simulink model "Primary_Arduino"  (R2018b)
settings: Solver=FixedStepAuto  StartTime=0  StopTime=300  MaxStep=0.01  RelTol=1e-4  EnableMultiTasking=on
libraries: pil_lib x1
settings Model: DataDictionary=data.sldd  Creator=Aliak  LastModifiedBy=Aliak
settings SolverCC: SolverResetMethod=Robust  MinimalZcImpactIntegration=on
settings OptimizationCC: DefaultParameterBehavior=Inlined  UseDivisionForNetSlopeComputation=on  UseFloatMulNetSlope=on  DefaultUnderspecifiedDataType=single  UseSpecifiedMinMax=on  InlineInvariantSignals=on  EnhancedBackFolding=on  BooleansAsBitfields=on  PassReuseOutputArgsAs=Individual arguments  StateBitsets=on  DataBitsets=on  ZeroExternalMemoryAtStartup=off  ZeroInternalMemoryAtStartup=off  NoFixptDivByZeroProtection=on  EfficientFloat2IntCast=on  LifeSpan=0.01  MaxStackSize=64  SimCompilerOptimization=on  OptimizeBlockOrder=speed  DifferentSizesBufferReuse=on
settings DebuggingCC: ConsistencyChecking=warning  ReadBeforeWriteMsg=DisableAll  WriteAfterWriteMsg=DisableAll  WriteAfterReadMsg=DisableAll  SolverPrmCheckMsg=warning  ParameterTunabilityLossMsg=error  UniqueDataStoreMsg=error  BusObjectLabelMismatch=error  StateNameClashWarn=warning  ForceCombineOutputUpdateInSim=on
settings HardwareCC: ProdBitPerInt=16  ProdBitPerPointer=16  ProdBitPerSizeT=16  ProdBitPerPtrDiffT=16  ProdLargestAtomicFloat=None  ProdWordSize=8  ProdLongLongMode=on  ProdHWDeviceType=Atmel->AVR
settings ModelReferenceCC: UpdateModelReferenceTargets=IfOutOfDate  EnableParallelModelReferenceBuilds=on  ModelReferenceMinAlgLoopOccurrences=on
settings SFSimCC: SimUserIncludeDirs="\"nativelibs/include\" \"nativelibs/src\" \"nativelibs/build\""  SFSimEcho=off  MATLABDynamicMemAlloc=off
settings RTWCC: SystemTargetFile=ert.tlc  HardwareBoard=Arduino Uno  TemplateMakefile=ert_default_tmf  GenerateReport=on  RTWUseSimCustomCode=on  CustomInclude="\"nativelibs/include\" \"nativelibs/src\" \"nativelibs/build\""  Toolchain=Arduino AVR  BuildConfiguration=Faster Runs  IncludeHyperlinkInReport=on  LaunchReport=on  PortableWordSizes=on  CreateSILPILBlock=PIL  GenerateTraceInfo=on  GenerateTraceReport=on  GenerateTraceReportSl=on  GenerateTraceReportSf=on  GenerateTraceReportEml=on  GenerateCodeMetricsReport=on
settings CodeAppCC: ForceParamTrailComments=on  IgnoreCustomStorageClasses=off  OperatorAnnotations=on  SimulinkDataObjDesc=on  SFDataObjDesc=on  CustomSymbolStrGlobalVar=rt$N$M  CustomSymbolStrType=$N$M  CustomSymbolStrFcn=$N$M$F  CustomSymbolStrMacro=$N$M  InsertBlockDesc=on
settings ERTTargetCC: TargetLangStandard=C99 (ISO)  UtilityFuncGeneration=Shared location  IncludeMdlTerminateFcn=off  CombineSignalStateStructs=on  SuppressErrorStatus=on  SupportNonFinite=off  SupportComplex=off  SupportVariableSizeSignals=on  CastingMode=Standards  ERTFilePackagingFormat=CompactWithDataFile

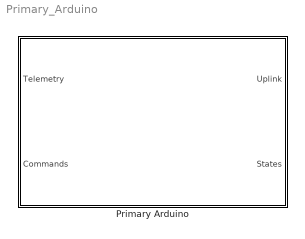
== system Primary_Arduino ==
  Primary Arduino : Subsystem  DialogController=pil_create_dialog  LoadFcn=|
      | try
      |    if ~strcmp(rtw.pil.getPILVersion, '9.5 (R2018b)_13')
      |       set_param(gcb, 'DialogController', '');
      |       set_param(gcb, 'DialogControllerArgs', '');
      |    end
      | catch e
      |       set_param(gcb, 'DialogController', '');
      |       set_param(gcb, 'DialogControllerArgs', '');
      | end
      mask help: PIL:pil:XILBlockMaskDesc
      mask Display: disp('PIL');

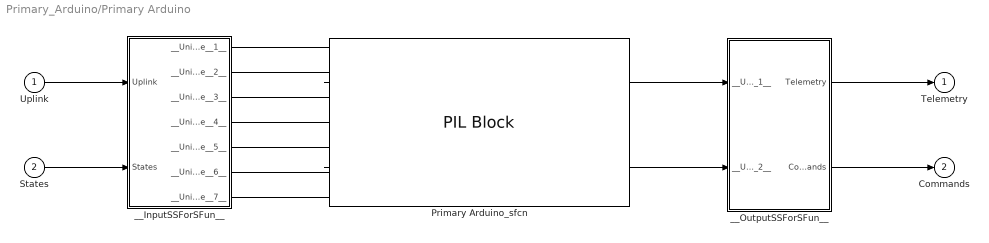
== system Primary_Arduino/Primary Arduino ==
  Uplink : Inport  OutDataTypeStr=Bus: Uplink
  States : Inport  Port=2
  Primary Arduino_sfcn : pil_lib/PIL Block  SimulationMode=PIL  IsTopModelPIL=off  CodeDir=D:\MATLABProjects\FEEG2001-FWUAV\Primary_ert_rtw  AnchorDir=D:\MATLABProjects\FEEG2001-FWUAV  ConfigName=Arduino Board  XrelIsTopModelCode=on  XrelIsReusable=off  XrelDWorkNames={}  XrelDWorkTypes={}  XrelModelArgVals={}  XrelOrderedParamNames={}
  __InputSSForSFun__ : Subsystem
  __OutputSSForSFun__ : Subsystem
  Telemetry : Outport  OutDataTypeStr=Bus: Sensors  SampleTime=[1 0]
  Commands : Outport  Port=2  OutDataTypeStr=Bus: Commands  SampleTime=[-1 0]
  wires:
  Uplink/1 -> __InputSSForSFun__/1(Uplink)
  States/1 -> __InputSSForSFun__/2(States)
  __InputSSForSFun__/1(__UniqueOutportName__1__) -> Primary Arduino_sfcn/1
  __InputSSForSFun__/2(__UniqueOutportName__2__) -> Primary Arduino_sfcn/2
  __InputSSForSFun__/3(__UniqueOutportName__3__) -> Primary Arduino_sfcn/3
  __InputSSForSFun__/4(__UniqueOutportName__4__) -> Primary Arduino_sfcn/4
  __InputSSForSFun__/5(__UniqueOutportName__5__) -> Primary Arduino_sfcn/5
  __InputSSForSFun__/6(__UniqueOutportName__6__) -> Primary Arduino_sfcn/6
  __InputSSForSFun__/7(__UniqueOutportName__7__) -> Primary Arduino_sfcn/7
  Primary Arduino_sfcn/1 -> __OutputSSForSFun__/1(__UniqueInportName__1__)
  Primary Arduino_sfcn/2 -> __OutputSSForSFun__/2(__UniqueInportName__2__)
  __OutputSSForSFun__/1(Telemetry) -> Telemetry/1
  __OutputSSForSFun__/2(Commands) -> Commands/1

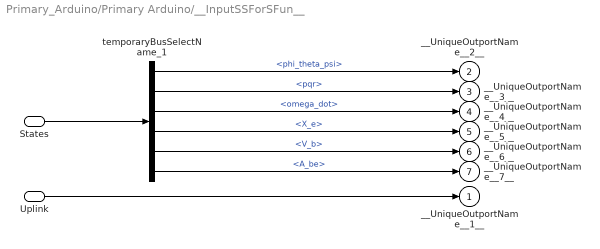
== system Primary_Arduino/Primary Arduino/__InputSSForSFun__ ==
  Uplink : Inport  OutDataTypeStr=Bus: Uplink
  States : Inport  Port=2
  temporaryBusSelectName_1 : BusSelector  OutputSignals=phi_theta_psi,pqr,omega_dot,X_e,V_b,A_be
  __UniqueOutportName__1__ : Outport
  __UniqueOutportName__2__ : Outport  Port=2
  __UniqueOutportName__3__ : Outport  Port=3
  __UniqueOutportName__4__ : Outport  Port=4
  __UniqueOutportName__5__ : Outport  Port=5
  __UniqueOutportName__6__ : Outport  Port=6
  __UniqueOutportName__7__ : Outport  Port=7
  wires:
  States/1 -> temporaryBusSelectName_1/1
  Uplink/1 -> __UniqueOutportName__1__/1
  temporaryBusSelectName_1/1 -> __UniqueOutportName__2__/1  "<phi_theta_psi>"
  temporaryBusSelectName_1/2 -> __UniqueOutportName__3__/1  "<pqr>"
  temporaryBusSelectName_1/3 -> __UniqueOutportName__4__/1  "<omega_dot>"
  temporaryBusSelectName_1/4 -> __UniqueOutportName__5__/1  "<X_e>"
  temporaryBusSelectName_1/5 -> __UniqueOutportName__6__/1  "<V_b>"
  temporaryBusSelectName_1/6 -> __UniqueOutportName__7__/1  "<A_be>"

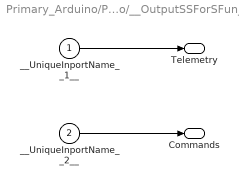
== system Primary_Arduino/Primary Arduino/__OutputSSForSFun__ ==
  __UniqueInportName__1__ : Inport
  __UniqueInportName__2__ : Inport  Port=2
  Telemetry : Outport  OutDataTypeStr=Bus: Sensors  SampleTime=[1 0]
  Commands : Outport  Port=2  OutDataTypeStr=Bus: Commands  SampleTime=[-1 0]
  wires:
  __UniqueInportName__1__/1 -> Telemetry/1
  __UniqueInportName__2__/1 -> Commands/1
